simulink model "control_model_landing"  (R2025b)
settings: Solver=VariableStepAuto  StartTime=0.0  StopTime=100  RelTol=1e-3
undefined symbols (not defined in the file): Am, B, Bm, Cm, Dm, engine_gimbal_speed, engine_max_angle, g, gain, initial_position, initial_rotation_speed, initial_teta, initial_velocity_x, initial_velocity_y, Iy, kd, kd_t, kp, kp_t, Kr, Kx, mass, max_thrust, P, static_margin, Xm
libraries: simulink_extras x7
settings Model: Creator=marti  LastModifiedBy=marti
settings DebuggingCC: AlgebraicLoopMsg=none

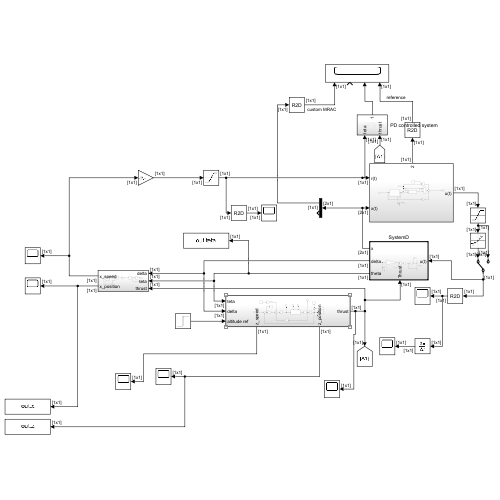
[thumbnail: Simulink's stored preview of the top-level diagram]
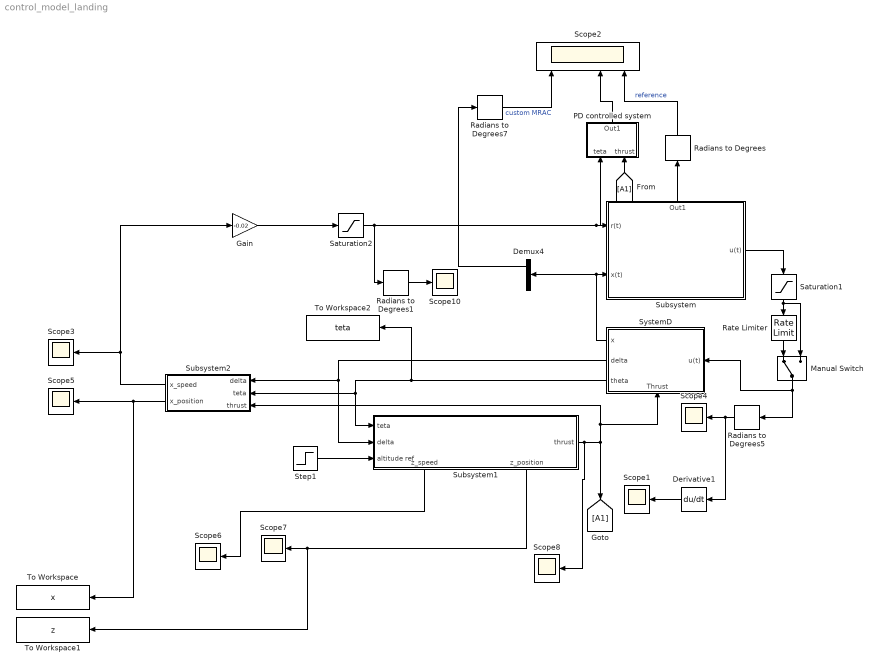
== system control_model_landing ==
  Demux4 : Demux  Outputs=2
  Derivative1 : Derivative
  Gain : Gain  Gain=-0.02
  Manual Switch : ManualSwitch
  PD controlled system : Subsystem
  Radians to Degrees{,1,5,7} (4 alike) : simulink_extras/Transformations/Radians to Degrees
  Rate Limiter : RateLimiter  RisingSlewLimit=engine_gimbal_speed  FallingSlewLimit=-engine_gimbal_speed  SampleTimeMode=inherited
  Saturation1 : Saturate  UpperLimit=engine_max_angle  LowerLimit=-engine_max_angle
  Saturation2 : Saturate  UpperLimit=abs(initial_teta)  LowerLimit=-abs(initial_teta)
  Scope{1,3..8,10} (8 alike) : Scope
      Scope1 settings: ActiveDisplayYMinimum=-28.142241468349347  ActiveDisplayYMaximum=25.537538650125914
      Scope10 settings: ActiveDisplayYMinimum=-22.045824307795336  ActiveDisplayYMaximum=2.44931155995471  DataLoggingVariableName=ScopeData2
      Scope3 settings: ActiveDisplayYMinimum=-5.0533475718137142  ActiveDisplayYMaximum=38.563721210831382  DataLoggingVariableName=ScopeData4
      Scope4 settings: ActiveDisplayYMinimum=-0.43563674490405779  ActiveDisplayYMaximum=0.51136704573008041  DataLoggingVariableName=ScopeData6
      Scope5 settings: ActiveDisplayYMinimum=-1  ActiveDisplayYMaximum=1  DataLoggingVariableName=ScopeData5
      Scope6 settings: ActiveDisplayYMinimum=-1  ActiveDisplayYMaximum=1  DataLoggingVariableName=ScopeData8
      Scope7 settings: ActiveDisplayYMinimum=-2.1390226252355866  ActiveDisplayYMaximum=7.7142899338381241  DataLoggingVariableName=ScopeData11
      Scope8 settings: ActiveDisplayYMinimum=-76.078081655342359  ActiveDisplayYMaximum=684.70273489808142  DataLoggingVariableName=ScopeData14
  Scope2 : Scope  NumInputPorts=4
      settings: ActiveDisplayYMinimum=-23.123538232771228  ActiveDisplayYMaximum=7.2037688134588285
  Step1 : Step  After=5  SampleTime=0
  Subsystem : Subsystem
      settings: PortSchema="{\"entries\":[{\"content\":{\"sides\":[{\"content\":{\"connectorIds\":[\"In1\",\"In2\"]},\"type\":\"ConnectorPlacement.EquallySpacedRectSide\",\"uuid\":\"2a5405b8-f474-466f-9064-f86b75893dd0\"},{\"content\":{\"connectorIds\":[\"Out1\"],\"side\":\"RIGHT\"},\"type\":\"ConnectorPlacement.EquallySpacedRectSide\",\"uuid\":\"ad673661-f4e9-494b-83cc-7452eec3fe31\"},{\"content\":{\"connectorIds\":[\"Out2\"],\"side\":\"TOP\"},\"type\":\"ConnectorPlacement.EquallySpacedRectSide\",\"uuid\":\"21a76317-3288-4ff3-bd02-68708e86e3a8\"}]},\"type\":\"ConnectorPlacement.EquallySpacedConnector\",\"uuid\":\"fc0ce599-928f-4c66-9629-0b98f2391e21\"}],\"packageUris\":[\"http://schema.mathworks.com/mf0/Connector/R2020b\"],\"version\":\"1.0\"}"
  Subsystem1 : Subsystem
      settings: PortSchema="{\"entries\":[{\"content\":{\"sides\":[{\"content\":{\"connectorIds\":[\"In1\",\"In2\",\"In3\"]},\"type\":\"ConnectorPlacement.EquallySpacedRectSide\",\"uuid\":\"5845fc2c-cfbe-4e3b-8b02-a8534e7ab1c9\"},{\"content\":{\"connectorIds\":[\"Out1\"],\"side\":\"RIGHT\"},\"type\":\"ConnectorPlacement.EquallySpacedRectSide\",\"uuid\":\"3881aa8e-ed7a-47ac-8b27-4b422192b2e5\"},{\"content\":{\"side\":\"TOP\"},\"type\":\"ConnectorPlacement.EquallySpacedRectSide\",\"uuid\":\"345c07f8-a317-4359-93cc-6a3e04a1c006\"},{\"content\":{\"connectorIds\":[\"Out2\",\"Out3\"],\"side\":\"BOTTOM\"},\"type\":\"ConnectorPlacement.EquallySpacedRectSide\",\"uuid\":\"ad64e6b9-582f-4f38-a8f0-c5fb38db2547\"}]},\"type\":\"ConnectorPlacement.EquallySpacedConnector\",\"uuid\":\"f5365408-e8d2-4396-a1e3-d7ed52685d7a\"}],\"packageUris\":[\"http://schema.mathworks.com/mf0/Connector/R2020b\"],\"version\":\"1.0\"}"
  Subsystem2 : Subsystem
  SystemD : Subsystem  TreatAsAtomicUnit=on
      settings: PortSchema="{\"entries\":[{\"content\":{\"sides\":[{\"content\":{\"connectorIds\":[\"In1\"]},\"type\":\"ConnectorPlacement.EquallySpacedRectSide\",\"uuid\":\"415d6c1e-0406-44b6-8f03-527b0a76a61e\"},{\"content\":{\"connectorIds\":[\"Out1\",\"Out2\",\"Out3\"],\"side\":\"RIGHT\"},\"type\":\"ConnectorPlacement.EquallySpacedRectSide\",\"uuid\":\"b01fbc7c-daf4-44fd-95a1-f9877c50f20d\"},{\"content\":{\"side\":\"TOP\"},\"type\":\"ConnectorPlacement.EquallySpacedRectSide\",\"uuid\":\"e1a1a26b-9f2a-40fe-9b8c-ace0723ba536\"},{\"content\":{\"connectorIds\":[\"In2\"],\"side\":\"BOTTOM\"},\"type\":\"ConnectorPlacement.EquallySpacedRectSide\",\"uuid\":\"cf849160-1adc-4083-9ccd-983d7a4d3225\"}]},\"type\":\"ConnectorPlacement.EquallySpacedConnector\",\"uuid\":\"7eec5b83-7b07-4bf0-a831-3aced5ecc844\"}],\"packageUris\":[\"http://schema.mathworks.com/mf0/Connector/R2020b\"],\"version\":\"1.0\"}"
  To Workspace : ToWorkspace  VariableName=x  SaveFormat=Timeseries  SampleTime=-1
  To Workspace1 : ToWorkspace  VariableName=z  SaveFormat=Timeseries  SampleTime=-1
  To Workspace2 : ToWorkspace  VariableName=teta  SaveFormat=Timeseries  SampleTime=-1
  wires:
  Subsystem/1(u(t)) -> Saturation1/1
  Radians to Degrees5/1 -> Scope4/1, Derivative1/1
  Radians to Degrees7/1 -> Scope2/1  "custom MRAC"
  Demux4/1 -> Radians to Degrees7/1
  Derivative1/1 -> Scope1/1
  SystemD/1(x) -> Demux4/1, Subsystem/2(x(t))
  Subsystem1/1(thrust) -> Scope8/1, Subsystem2/3(thrust), SystemD/2(Thrust), [A1]
  SystemD/3(theta) -> To Workspace2/1, Subsystem2/2(teta), Subsystem1/1(teta)
  Subsystem/2(Out1) -> Radians to Degrees/1
  PD controlled system/1(Out1) -> Scope2/3
  Radians to Degrees/1 -> Scope2/4  "reference"
  [A1] -> PD controlled system/2(thrust)
  SystemD/2(delta) -> Subsystem2/1(delta), Subsystem1/2(delta)
  Subsystem2/1(x_speed) -> Gain/1, Scope3/1
  Subsystem2/2(x_position) -> To Workspace/1, Scope5/1
  Subsystem1/2(z_speed) -> Scope6/1
  Subsystem1/3(z_position) -> To Workspace1/1, Scope7/1
  Radians to Degrees1/1 -> Scope10/1
  Gain/1 -> Saturation2/1
  Saturation2/1 -> PD controlled system/1(teta), Subsystem/1(r(t)), Radians to Degrees1/1
  Step1/1 -> Subsystem1/3(altitude ref)
  Saturation1/1 -> Manual Switch/2, Rate Limiter/1
  Rate Limiter/1 -> Manual Switch/1
  Manual Switch/1 -> SystemD/1(u(t)), Radians to Degrees5/1

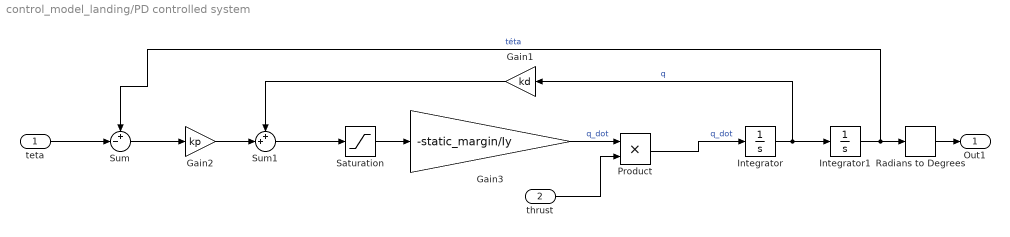
== system control_model_landing/PD controlled system ==
  teta : Inport
  thrust : Inport  Port=2
  Gain1 : Gain  Gain=kd
  Gain2 : Gain  Gain=kp
  Gain3 : Gain  Gain=-static_margin/Iy
  Integrator : Integrator  InitialCondition=initial_rotation_speed
  Integrator1 : Integrator  InitialCondition=initial_teta
  Product : Product
  Radians to Degrees : simulink_extras/Transformations/Radians to Degrees
  Saturation : Saturate  UpperLimit=engine_max_angle  LowerLimit=-engine_max_angle
  Sum : Sum  Inputs=+-|
  Sum1 : Sum  Inputs=++|
  Out1 : Outport
  wires:
  Integrator/1 -> Gain1/1, Integrator1/1  "q"
  Gain3/1 -> Product/1  "q_dot"
  thrust/1 -> Product/2
  Gain2/1 -> Sum1/2
  Product/1 -> Integrator/1  "q_dot"
  Sum1/1 -> Saturation/1
  Saturation/1 -> Gain3/1
  Gain1/1 -> Sum1/1
  Integrator1/1 -> Radians to Degrees/1, Sum/1  "téta"
  Sum/1 -> Gain2/1
  teta/1 -> Sum/2
  Radians to Degrees/1 -> Out1/1

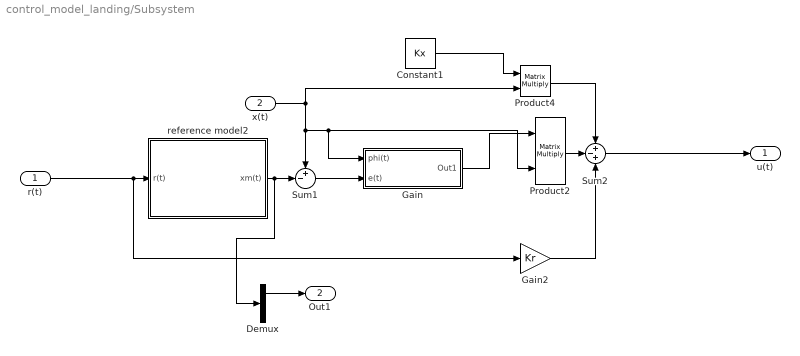
== system control_model_landing/Subsystem ==
  r(t) : Inport
  x(t) : Inport  Port=2  PortDimensions=[2 1]
  Constant1 : Constant  Value=Kx  VectorParams1D=off
  Demux : Demux  Outputs=2
  Gain : Subsystem
  Gain2 : Gain  Gain=Kr
  Product2 : Product  Multiplication=Matrix(*)
  Product4 : Product  Multiplication=Matrix(*)
  Sum1 : Sum  Inputs=+-|
  Sum2 : Sum  Inputs=+-+
  reference model2 : Subsystem  TreatAsAtomicUnit=on
  u(t) : Outport
  Out1 : Outport  Port=2
  wires:
  r(t)/1 -> Gain2/1, reference model2/1(r(t))
  reference model2/1(xm(t)) -> Demux/1, Sum1/2
  x(t)/1 -> Product4/2, Product2/2, Gain/1(phi(t)), Sum1/1
  Product2/1 -> Sum2/2
  Sum1/1 -> Gain/2(e(t))
  Constant1/1 -> Product4/1
  Product4/1 -> Sum2/1
  Gain2/1 -> Sum2/3
  Sum2/1 -> u(t)/1
  Gain/1(Out1) -> Product2/1
  Demux/1 -> Out1/1

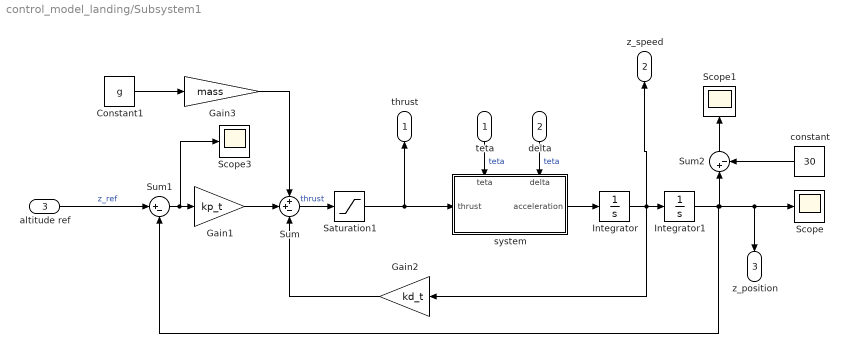
== system control_model_landing/Subsystem1 ==
  teta : Inport
  delta : Inport  Port=2
  altitude ref : Inport  Port=3
  Constant1 : Constant  Value=g
  Gain1 : Gain  Gain=kp_t
  Gain2 : Gain  Gain=kd_t
  Gain3 : Gain  Gain=mass
  Integrator : Integrator  InitialCondition=initial_velocity_y
  Integrator1 : Integrator  InitialCondition=initial_position
  Saturation1 : Saturate  UpperLimit=max_thrust  LowerLimit=0
  Scope : Scope
      settings: ActiveDisplayYMinimum=-203.34625268465874  ActiveDisplayYMaximum=578.14958363162873  DataLoggingVariableName=ScopeData7
  Scope1 : Scope
      settings: ActiveDisplayYMinimum=-59.812619871124554  ActiveDisplayYMaximum=528.86806887456942  DataLoggingVariableName=ScopeData9
  Scope3 : Scope
      settings: ActiveDisplayYMinimum=-1  ActiveDisplayYMaximum=1  DataLoggingVariableName=ScopeData10
  Sum : Sum  Inputs=++-
  Sum1 : Sum  Inputs=|+-
  Sum2 : Sum  Inputs=|+-
  constant : Constant  Value=30
  system : Subsystem
      settings: PortSchema="{\"entries\":[{\"content\":{\"sides\":[{\"content\":{\"connectorIds\":[\"In1\"]},\"type\":\"ConnectorPlacement.EquallySpacedRectSide\",\"uuid\":\"38ff2807-5c3f-4880-9c07-8b6447135695\"},{\"content\":{\"connectorIds\":[\"Out1\"],\"side\":\"RIGHT\"},\"type\":\"ConnectorPlacement.EquallySpacedRectSide\",\"uuid\":\"bc1e5b06-9245-4ba5-abe1-979ca83ec99f\"},{\"content\":{\"connectorIds\":[\"In2\",\"In3\"],\"side\":\"TOP\"},\"type\":\"ConnectorPlacement.EquallySpacedRectSide\",\"uuid\":\"205a83f4-1465-412a-8e3f-6475f5e18be2\"}]},\"type\":\"ConnectorPlacement.EquallySpacedConnector\",\"uuid\":\"dff9f67b-b046-4801-81e2-6dc88e83eb4a\"}],\"packageUris\":[\"http://schema.mathworks.com/mf0/Connector/R2020b\"],\"version\":\"1.0\"}"
  thrust : Outport
  z_speed : Outport  Port=2
  z_position : Outport  Port=3
  wires:
  system/1(acceleration) -> Integrator/1
  Integrator1/1 -> z_position/1, Scope/1, Sum2/1, Sum1/2
  Gain1/1 -> Sum/2
  Gain2/1 -> Sum/3
  Sum/1 -> Saturation1/1  "thrust"
  Sum1/1 -> Scope3/1, Gain1/1
  Integrator/1 -> z_speed/1, Integrator1/1, Gain2/1
  Gain3/1 -> Sum/1
  Constant1/1 -> Gain3/1
  Saturation1/1 -> system/1(thrust), thrust/1
  altitude ref/1 -> Sum1/1  "z_ref"
  teta/1 -> system/2(teta)  "teta"
  constant/1 -> Sum2/2
  Sum2/1 -> Scope1/1
  delta/1 -> system/3(delta)  "teta"

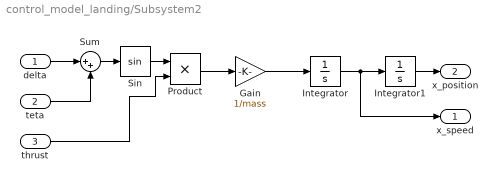
== system control_model_landing/Subsystem2 ==
  delta : Inport
  teta : Inport  Port=2
  thrust : Inport  Port=3
  Gain : Gain  Gain=1/mass
  Integrator : Integrator  InitialCondition=initial_velocity_x
  Integrator1 : Integrator  InitialCondition=1
  Product : Product
  Sin : Trigonometry
  Sum : Sum  Inputs=|++
  x_speed : Outport
  x_position : Outport  Port=2
  wires:
  delta/1 -> Sum/1
  teta/1 -> Sum/2
  Sum/1 -> Sin/1
  Sin/1 -> Product/1
  thrust/1 -> Product/2
  Product/1 -> Gain/1
  Gain/1 -> Integrator/1
  Integrator/1 -> x_speed/1, Integrator1/1
  Integrator1/1 -> x_position/1

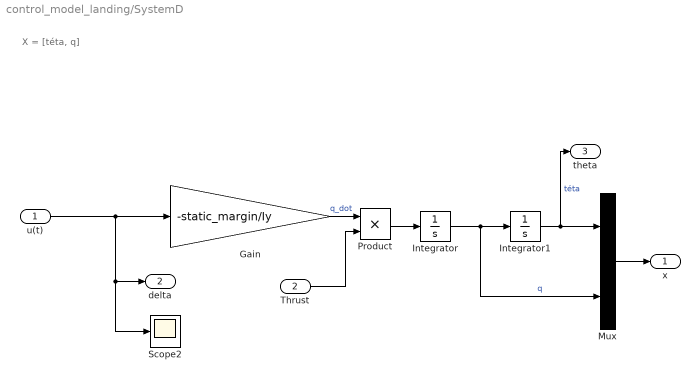
== system control_model_landing/SystemD ==
  note: X = [téta, q]
  u(t) : Inport
  Thrust : Inport  Port=2
  Gain : Gain  Gain=-static_margin/Iy
  Integrator : Integrator  InitialCondition=initial_rotation_speed
  Integrator1 : Integrator  InitialCondition=initial_teta
  Mux : Mux  Inputs=2
  Product : Product
  Scope2 : Scope
      settings: ActiveDisplayYMinimum=-1  ActiveDisplayYMaximum=1  DataLoggingVariableName=ScopeData3
  x : Outport
  delta : Outport  Port=2
  theta : Outport  Port=3
  wires:
  Integrator/1 -> Integrator1/1, Mux/2  "q"
  Integrator1/1 -> theta/1, Mux/1  "téta"
  Mux/1 -> x/1
  u(t)/1 -> Scope2/1, delta/1, Gain/1
  Gain/1 -> Product/1  "q_dot"
  Product/1 -> Integrator/1
  Thrust/1 -> Product/2

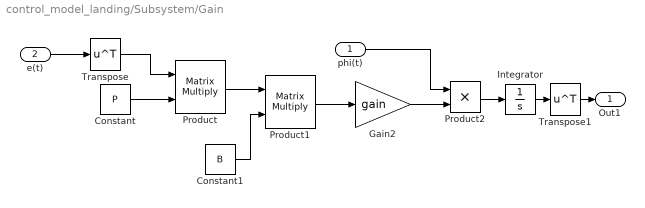
== system control_model_landing/Subsystem/Gain ==
  phi(t) : Inport
  e(t) : Inport  Port=2
  Constant : Constant  Value=P  VectorParams1D=off
  Constant1 : Constant  Value=B  VectorParams1D=off
  Gain2 : Gain  Gain=gain
  Integrator : Integrator
  Product : Product  Multiplication=Matrix(*)
  Product1 : Product  Multiplication=Matrix(*)
  Product2 : Product
  Transpose : Math  Operator=transpose
  Transpose1 : Math  Operator=transpose
  Out1 : Outport
  wires:
  Product1/1 -> Gain2/1
  phi(t)/1 -> Product2/1
  Product/1 -> Product1/1
  Constant1/1 -> Product1/2
  Gain2/1 -> Product2/2
  e(t)/1 -> Transpose/1
  Constant/1 -> Product/2
  Transpose/1 -> Product/1
  Product2/1 -> Integrator/1
  Integrator/1 -> Transpose1/1
  Transpose1/1 -> Out1/1

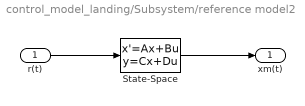
== system control_model_landing/Subsystem/reference model2 ==
  r(t) : Inport
  State-Space : StateSpace  A=Am  B=Bm  C=Cm  D=Dm  InitialCondition=Xm
  xm(t) : Outport  PortDimensions=[2 1]
  wires:
  State-Space/1 -> xm(t)/1
  r(t)/1 -> State-Space/1

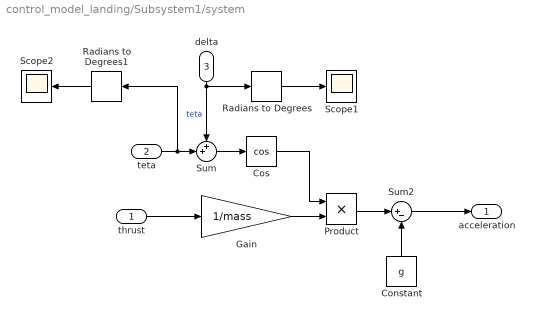
== system control_model_landing/Subsystem1/system ==
  thrust : Inport
  teta : Inport  Port=2
  delta : Inport  Port=3
  Constant : Constant  Value=g
  Cos : Trigonometry  Operator=cos
  Gain : Gain  Gain=1/mass
  Product : Product
  Radians to Degrees : simulink_extras/Transformations/Radians to Degrees
  Radians to Degrees1 : simulink_extras/Transformations/Radians to Degrees
  Scope1 : Scope
      settings: ActiveDisplayYMinimum=-1  ActiveDisplayYMaximum=1  DataLoggingVariableName=ScopeData12
  Scope2 : Scope
      settings: ActiveDisplayYMinimum=-1  ActiveDisplayYMaximum=1  DataLoggingVariableName=ScopeData13
  Sum : Sum  Inputs=++|
  Sum2 : Sum  Inputs=|+-
  acceleration : Outport
  wires:
  Constant/1 -> Sum2/2
  Sum2/1 -> acceleration/1
  thrust/1 -> Gain/1
  Gain/1 -> Product/2
  Product/1 -> Sum2/1
  Cos/1 -> Product/1
  teta/1 -> Radians to Degrees1/1, Sum/2
  delta/1 -> Sum/1, Radians to Degrees/1  "teta"
  Sum/1 -> Cos/1
  Radians to Degrees/1 -> Scope1/1
  Radians to Degrees1/1 -> Scope2/1
